simulink model "variable"  (R2024b)
settings: Solver=FixedStepDiscrete  StartTime=0.0  StopTime=20  RelTol=1e-3  EnableMultiTasking=on
libraries: simulink x3
settings Model: ModifiedByFormat=The MathWorks, Inc.  Creator=The MathWorks, Inc.  LastModifiedBy=The MathWorks, Inc.
settings SolverCC: AlgebraicLoopSolver=TrustRegion
settings DataIOCC: LimitDataPoints=on  SaveFormat=Array
settings OptimizationCC: ReuseModelBlockBuffer=off  ExpressionDepthLimit=2147483647  InitFltsAndDblsToZero=on  LifeSpan=inf
settings DebuggingCC: SolverPrmCheckMsg=warning  FcnCallInpInsideContextMsg=warning  UnconnectedInputMsg=warning  UnconnectedOutputMsg=warning  UnconnectedLineMsg=warning  AllowSymbolicDim=off  StateNameClashWarn=warning  SFUnexpectedBacktrackingDiag=warning  SFNoUnconditionalDefaultTransitionDiag=warning  SFExecutionAtInitializationDiag=none  ArithmeticOperatorsInVariantConditions=warning
settings HardwareCC: ProdBitPerPointer=32  ProdBitPerSizeT=32  ProdBitPerPtrDiffT=32  ProdLargestAtomicFloat=None  ProdIntDivRoundTo=Undefined  ProdEndianess=Unspecified  ProdWordSize=32  ProdHWDeviceType=32-bit Generic
settings ModelReferenceCC: EnableRefExpFcnMdlSchedulingChecks=on  PropagateSignalLabelsOutOfModel=off
settings SFSimCC: SimUseLocalCustomCode=off  SimParseCustomCode=off  CustomCodeUndefinedFunction=UseInterfaceOnly
settings RTWCC: RTWUseLocalCustomCode=off  GPUComputeCapability=3.5  DLArmComputeVersion=19.05
settings CodeAppCC: StateflowObjectComments=on
settings GRTTargetCC: TargetLangStandard=C89/C90 (ANSI)  CombineOutputUpdateFcns=off  GRTInterface=on
settings ConfigComp: CovMetricSettings=dw  CovSaveCumulativeToWorkspaceVar=on  CovSaveSingleToWorkspaceVar=on  CovExternalEMLEnable=off

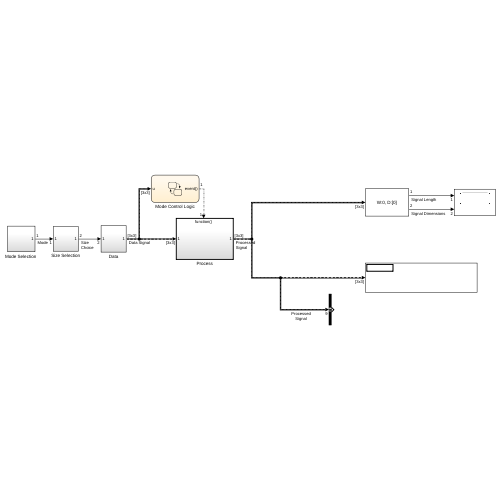
[thumbnail: Simulink's stored preview of the top-level diagram]
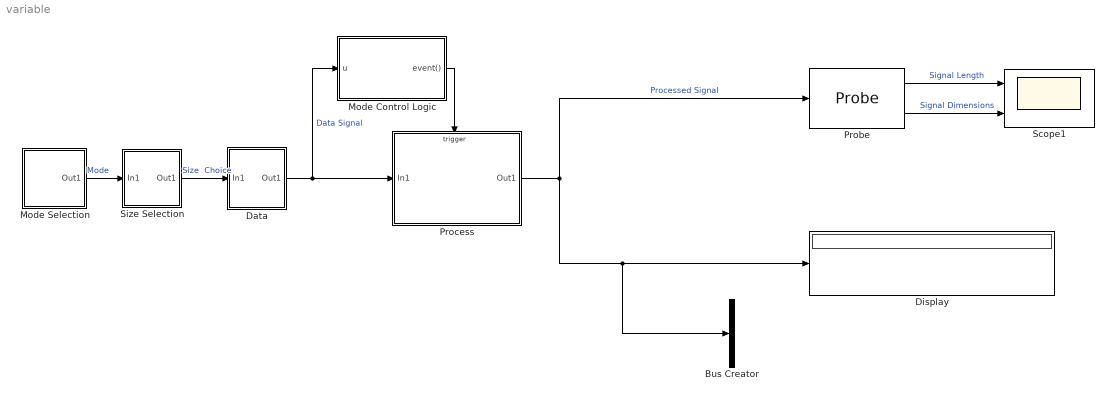
== system variable ==
  Bus Creator : BusCreator  Inputs=1  OutDataTypeStr=Bus: BusObject  NonVirtualBus=on
      settings: InheritFromInputs=off
  Data : Subsystem
  Display : Display
  Mode Control Logic : Stateflow chart  TreatAsAtomicUnit=on
  "Mode Selection " : Subsystem
  Probe : Probe  ProbeSampleTime=off  ProbeComplexSignal=off  ProbeSignalDimensions=on
  Process : Subsystem  TreatAsAtomicUnit=on
  Scope1 : Scope  NumInputPorts=2
  Size Selection : Subsystem
  wires:
  Data/1(Out1) -> Process/1(In1), Mode Control Logic/1(u)  "Data Signal"
  "Mode Selection "/1(Out1) -> Size Selection/1(In1)  "Mode"
  Size Selection/1(Out1) -> Data/1(In1)  "Size  Choice"
  Probe/1 -> Scope1/1  "Signal Length"
  Mode Control Logic/1(event()) -> Process/Trigger
  Probe/2 -> Scope1/2  "Signal Dimensions"
  Process/1(Out1) -> Bus Creator/1, Display/1, Probe/1  "Processed Signal"

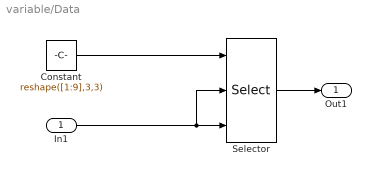
== system variable/Data ==
  In1 : Inport
  Constant : Constant  Value=reshape([1:9],3,3)
  Selector : Selector  NumberOfDimensions=2  InputPortWidth=3  IndexOptions=Starting and ending indices (port),Starting and ending indices (port)  Indices=[1 3],1  OutputSizes=1,1
  Out1 : Outport  VectorParamsAs1DForOutWhenUnconnected=off
  wires:
  Constant/1 -> Selector/1
  Selector/1 -> Out1/1
  In1/1 -> Selector/3, Selector/2

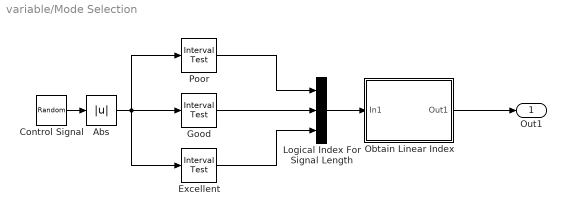
== system variable/Mode Selection  ==
  Abs : Abs  SaturateOnIntegerOverflow=off
  Control Signal : RandomNumber  Variance=0.25  SampleTime=1
  Excellent : simulink/Logic and Bit Operations/Interval Test  IntervalClosedRight=off  uplimit=inf  IntervalClosedLeft=on  lowlimit=0.50  OutDataTypeStr=uint8
  Good : simulink/Logic and Bit Operations/Interval Test  IntervalClosedRight=off  uplimit=0.50  IntervalClosedLeft=on  lowlimit=0.25  OutDataTypeStr=uint8
  Logical Index For Signal Length : Concatenate  NumInputs=3
  Obtain Linear Index : Subsystem
  Poor : simulink/Logic and Bit Operations/Interval Test  IntervalClosedRight=off  uplimit=0.25  IntervalClosedLeft=on  lowlimit=0.0  OutDataTypeStr=uint8
  Out1 : Outport  VectorParamsAs1DForOutWhenUnconnected=off
  wires:
  Logical Index For Signal Length/1 -> Obtain Linear Index/1(In1)
  Poor/1 -> Logical Index For Signal Length/1
  Excellent/1 -> Logical Index For Signal Length/3
  Good/1 -> Logical Index For Signal Length/2
  Abs/1 -> Excellent/1, Poor/1, Good/1
  Obtain Linear Index/1(Out1) -> Out1/1
  Control Signal/1 -> Abs/1

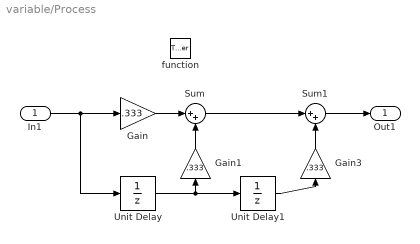
== system variable/Process ==
  In1 : Inport
  function : TriggerPort  TriggerType=function-call  VariantControl=(inherit)  StatesWhenEnabling=reset  PropagateVarSize=Only when enabling  SampleTimeType=periodic
  Gain : Gain  Gain=.333
  Gain1 : Gain  Gain=.333
  Gain3 : Gain  Gain=.333
  Sum : Sum  Inputs=|++
  Sum1 : Sum  Inputs=|++
  Unit Delay : UnitDelay  SampleTime=-1  HasFrameUpgradeWarning=on
  Unit Delay1 : UnitDelay  SampleTime=-1  HasFrameUpgradeWarning=on
  Out1 : Outport  VectorParamsAs1DForOutWhenUnconnected=off
  wires:
  Unit Delay/1 -> Gain1/1, Unit Delay1/1
  Gain/1 -> Sum/1
  Gain1/1 -> Sum/2
  In1/1 -> Gain/1, Unit Delay/1
  Unit Delay1/1 -> Gain3/1
  Gain3/1 -> Sum1/2
  Sum/1 -> Sum1/1
  Sum1/1 -> Out1/1

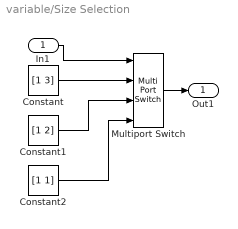
== system variable/Size Selection ==
  In1 : Inport
  Constant : Constant  Value=[1 3]
  Constant1 : Constant  Value=[1 2]
  Constant2 : Constant  Value=[1 1]
  Multiport Switch : MultiPortSwitch  SaturateOnIntegerOverflow=off  InputSameDT=off
  Out1 : Outport  VectorParamsAs1DForOutWhenUnconnected=off
  wires:
  Constant/1 -> Multiport Switch/2
  Constant1/1 -> Multiport Switch/3
  Constant2/1 -> Multiport Switch/4
  In1/1 -> Multiport Switch/1
  Multiport Switch/1 -> Out1/1

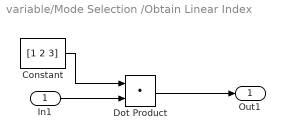
== system variable/Mode Selection /Obtain Linear Index ==
  In1 : Inport
  Constant : Constant  Value=[1 2 3]
  Dot Product : DotProduct  InputSameDT=off  OutDataTypeStr=Inherit: Inherit via internal rule
  Out1 : Outport  VectorParamsAs1DForOutWhenUnconnected=off
  wires:
  Constant/1 -> Dot Product/1
  Dot Product/1 -> Out1/1
  In1/1 -> Dot Product/2

== stateflow chart variable/Mode Control Logic ==
  settings: updateMethod=DISCRETE  sampleTime=1
  state S
    entry: event;
    during: event;
    bind: event
  (default) -> S
  S -> S : [size_detect()]
  data: y function_output double; u input
  events: event output FUNCTION_CALL_EVENT
  function y = size_detect:
    | function y = size_detect
    | % Detect signal size changes.
    | % When the input signal size changes the output is set to 1, otherwise it 
    | % is 0.
    | 
    | persistent prevSize;
    | 
    | if isempty(prevSize)
    |    prevSize = 0; 
    | end
    | 
    | if length(u(:)) ~= prevSize
    |     prevSize = length(u(:));
    |     y = 1;
    | else
    |     y = 0;
    | end
